simulink model "KinematicsCheck"  (R2017a)
settings: Solver=VariableStepAuto  StartTime=0.0  StopTime=10.0  RelTol=1e-3
libraries: simulink x5
settings Model: Creator=Matthew  LastModifiedBy=Matthew

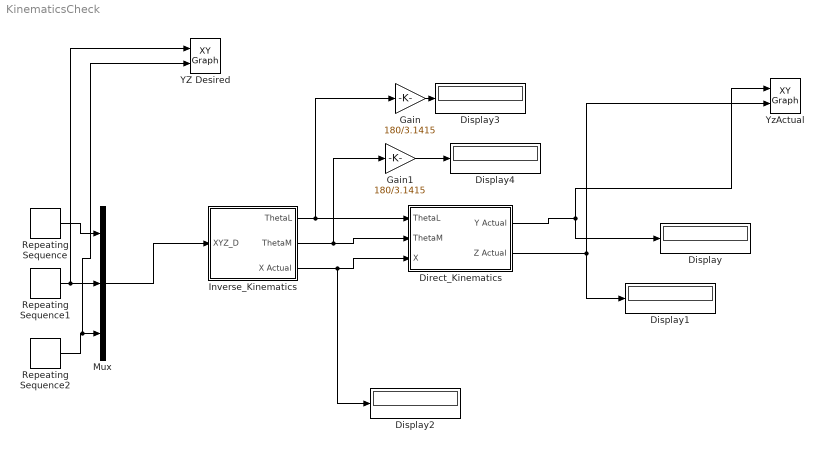
== system KinematicsCheck ==
  Direct_Kinematics : Subsystem
  Display{,1..4} (5 alike) : Display
  Gain : Gain  Gain=180/3.1415
  Gain1 : Gain  Gain=180/3.1415
  "Inverse_Kinematics " : Subsystem
  Mux : Mux  Inputs=3
  Repeating Sequence : simulink/Sources/Repeating Sequence  rep_seq_t=[1,2,3,4,5,6,7,8,9]  rep_seq_y=ones(9,1)*10
  Repeating Sequence1 : simulink/Sources/Repeating Sequence  rep_seq_t=[1,2,3,4,5,6,7,8,9]  rep_seq_y=[1,2,3,4,5,6,7,8,9]
  Repeating Sequence2 : simulink/Sources/Repeating Sequence  rep_seq_t=[1,2,3,4,5,6,7,8,9]  rep_seq_y=[1,2,3,4,5,6,7,8,9]
  YZ Desired : simulink/Sinks/XY Graph  xmin=-15  xmax=15  ymin=-15  ymax=15  st=0.1
  "YzActual " : simulink/Sinks/XY Graph  xmin=-15  xmax=15  ymin=-15  ymax=15  st=0.1
  wires:
  "Inverse_Kinematics "/3("X Actual ") -> Direct_Kinematics/3("X "), Display2/1
  "Inverse_Kinematics "/2("ThetaM ") -> Direct_Kinematics/2(ThetaM), Gain1/1
  "Inverse_Kinematics "/1(ThetaL) -> Direct_Kinematics/1("ThetaL "), Gain/1
  Gain/1 -> Display3/1
  Gain1/1 -> Display4/1
  Direct_Kinematics/1("Y Actual ") -> "YzActual "/1, Display/1
  Direct_Kinematics/2(Z Actual) -> Display1/1, "YzActual "/2
  Repeating Sequence1/1 -> YZ Desired/1, Mux/2
  Repeating Sequence/1 -> Mux/1
  Repeating Sequence2/1 -> YZ Desired/2, Mux/3
  Mux/1 -> "Inverse_Kinematics "/1(XYZ_D)

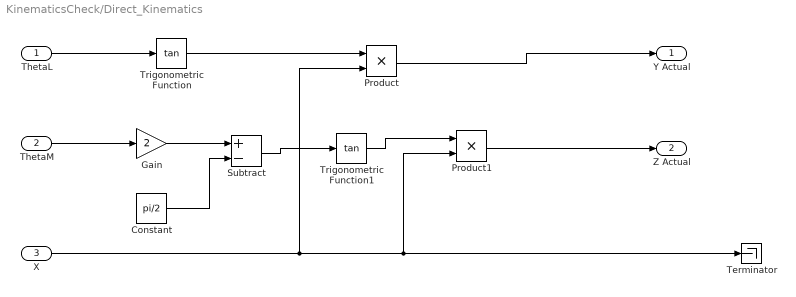
== system KinematicsCheck/Direct_Kinematics ==
  "ThetaL " : Inport
  ThetaM : Inport  Port=2
  "X " : Inport  Port=3
  Constant : Constant  Value=pi/2
  Gain : Gain  Gain=2
  Product : Product
  Product1 : Product
  Subtract : Sum  Inputs=+-
  Terminator : Terminator
  Trigonometric Function : Trigonometry  Operator=tan  ApproximationMethod=CORDIC  NumberOfIterations=1
  Trigonometric Function1 : Trigonometry  Operator=tan  ApproximationMethod=CORDIC  NumberOfIterations=1
  "Y Actual " : Outport
  Z Actual : Outport  Port=2
  wires:
  "ThetaL "/1 -> Trigonometric Function/1
  Trigonometric Function/1 -> Product/1
  "X "/1 -> Product/2, Product1/2, Terminator/1
  Product/1 -> "Y Actual "/1
  Constant/1 -> Subtract/2
  ThetaM/1 -> Gain/1
  Gain/1 -> Subtract/1
  Subtract/1 -> Trigonometric Function1/1
  Trigonometric Function1/1 -> Product1/1
  Product1/1 -> Z Actual/1

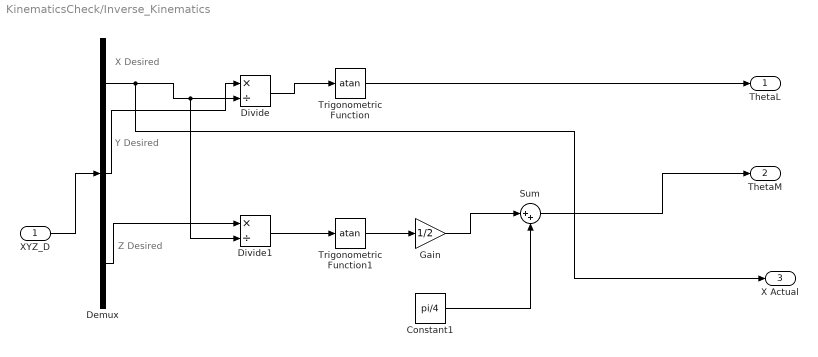
== system KinematicsCheck/Inverse_Kinematics  ==
  note: Z Desired
  note: Y Desired
  note: X Desired
  XYZ_D : Inport
  Constant1 : Constant  Value=pi/4
  Demux : Demux  Outputs=3
  Divide : Product  Inputs=*/
  Divide1 : Product  Inputs=*/
  Gain : Gain  Gain=1/2
  Sum : Sum  Inputs=|++
  Trigonometric Function : Trigonometry  Operator=atan
  Trigonometric Function1 : Trigonometry  Operator=atan
  ThetaL : Outport
  "ThetaM " : Outport  Port=2
  "X Actual " : Outport  Port=3
  wires:
  XYZ_D/1 -> Demux/1
  Demux/2 -> Divide/1
  Demux/1 -> "X Actual "/1, Divide1/2, Divide/2
  Divide/1 -> Trigonometric Function/1
  Trigonometric Function/1 -> ThetaL/1
  Demux/3 -> Divide1/1
  Divide1/1 -> Trigonometric Function1/1
  Constant1/1 -> Sum/2
  Sum/1 -> "ThetaM "/1
  Trigonometric Function1/1 -> Gain/1
  Gain/1 -> Sum/1
